simulink model "variable_delay_echo"  (R2020b)
settings: Solver=FixedStepDiscrete  StartTime=0.0  StopTime=stopTime  RelTol=1e-3
InitFcn:
  | initCallback
StopFcn:
  | stopCallback
values from neighbouring files (symbols this model uses):
  mp = sm_init_avalon_signals(mp)    [sm_callback_init.m]    (also in sm_callback_stop.m = sm_stop_verify(mp))
settings Model: Creator=Ross  LastModifiedBy=wickh
settings SolverCC: MinimalZcImpactIntegration=on
settings DataIOCC: ReturnWorkspaceOutputs=off
settings OptimizationCC: DefaultParameterBehavior=Inlined
settings DebuggingCC: ReadBeforeWriteMsg=DisableAll  WriteAfterWriteMsg=DisableAll  WriteAfterReadMsg=DisableAll  AlgebraicLoopMsg=error  MultiTaskDSMMsg=none  SingleTaskRateTransMsg=error  PregeneratedLibrarySubsystemCodeDiagnostic=none  ArithmeticOperatorsInVariantConditions=warning
settings HardwareCC: ProdBitPerPointer=32  ProdBitPerSizeT=32  ProdBitPerPtrDiffT=32  ProdLargestAtomicFloat=None  ProdIntDivRoundTo=Undefined  ProdEndianess=Unspecified  ProdWordSize=32  ProdHWDeviceType=ASIC/FPGA->ASIC/FPGA  TargetBitPerPointer=64  TargetBitPerSizeT=64  TargetBitPerPtrDiffT=64  TargetLongLongMode=on  TargetIntDivRoundTo=Zero  TargetEndianess=LittleEndian  TargetWordSize=64  TargetHWDeviceType=Custom Processor->MATLAB Host Computer  ProdEqTarget=off
settings ModelReferenceCC: UpdateModelReferenceTargets=IfOutOfDate
settings SFSimCC: SFSimEcho=off  SimUseLocalCustomCode=off  CustomCodeUndefinedFunction=UseInterfaceOnly
settings RTWCC: RTWUseLocalCustomCode=off

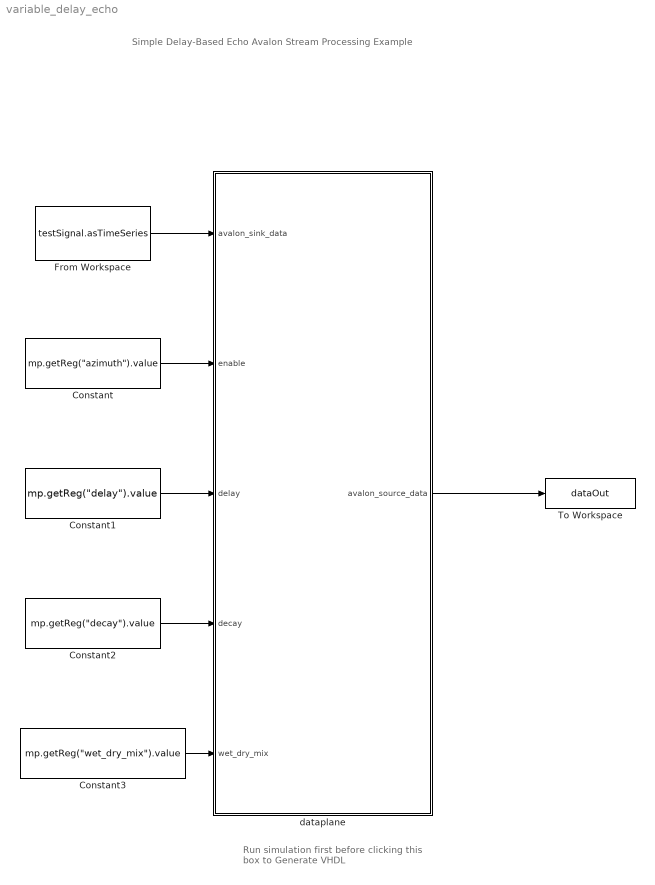
== system variable_delay_echo ==
  note: Simple Delay-Based Echo
      | Avalon Stream Processing Example
  note: Run simulation first
      | before clicking this box to
      | Generate VHDL
  Constant : Constant  Value="mp.getReg(\"azimuth\").value"  SampleTime=-1
  Constant1 : Constant  Value="mp.getReg(\"delay\").value"  SampleTime=-1
  Constant2 : Constant  Value="mp.getReg(\"decay\").value"  SampleTime=-1
  Constant3 : Constant  Value="mp.getReg(\"wet_dry_mix\").value"  SampleTime=-1
  From Workspace : FromWorkspace  VariableName=testSignal.asTimeSeries  SampleTime=mp.Ts_sim  OutputAfterFinalValue=Setting to zero
  To Workspace : ToWorkspace  VariableName=dataOut  SaveFormat=Timeseries  SampleTime=-1
  dataplane : Subsystem  TreatAsAtomicUnit=on
  wires:
  From Workspace/1 -> dataplane/1(avalon_sink_data)
  dataplane/1(avalon_source_data) -> To Workspace/1
  Constant2/1 -> dataplane/4(decay)
  Constant3/1 -> dataplane/5(wet_dry_mix)
  Constant1/1 -> dataplane/3(delay)
  Constant/1 -> dataplane/2(enable)

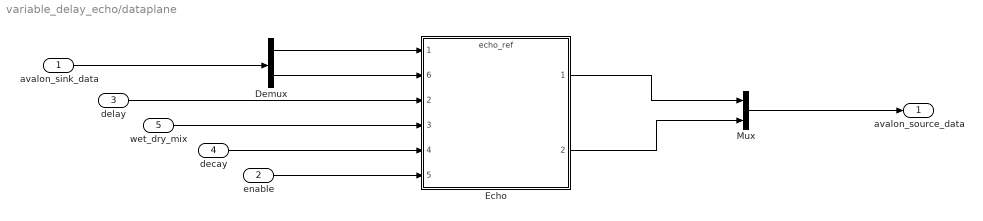
== system variable_delay_echo/dataplane ==
  avalon_sink_data : Inport
  enable : Inport  Port=2
  delay : Inport  Port=3
  decay : Inport  Port=4
  wet_dry_mix : Inport  Port=5
  Demux : Demux  Outputs=2
  Echo : ModelReference  ModelNameDialog=echo_ref  SimulationMode=Normal  ModelReferenceVersion=1.168
      settings: PortSchema="{\"entries\":[{\"content\":{\"sides\":[{\"content\":{\"connectorIds\":[\"In1\",\"In6\",\"In2\",\"In3\",\"In4\",\"In5\"]},\"type\":\"ConnectorPlacement.EquallySpacedRectSide\",\"uuid\":\"e306e1ad-d1b8-4582-952d-4c4191a99a81\"},{\"content\":{\"connectorIds\":[\"Out1\",\"Out2\"],\"side\":\"RIGHT\"},\"type\":\"ConnectorPlacement.EquallySpacedRectSide\",\"uuid\":\"8133f08a-39d0-44da-b52e-b96b1c72783c\"},{\"content\":{\"connectorIds\":[],\"side\":\"TOP\"},\"type\":\"ConnectorPlacement.EquallySpacedRectSide\",\"uuid\":\"327e31c7-8f91-4124-82a4-b2c62ce56765\"},{\"content\":{\"connectorIds\":[],\"side\":\"HIDDEN\"},\"type\":\"ConnectorPlacement.EquallySpacedRectSide\",\"uuid\":\"f85fe833-603d-4d04-9a61-60dde0930239\"}]},\"type\":\"ConnectorPlacement.EquallySpacedConnector\",\"uuid\":\"c6b2a458-4634-4ce8-98bc-50a2a0ff1bc4\"}],\"packageUris\":[\"http://schema.mathworks.com/mf0/Connector/R2020b\"],\"version\":\"1.0\"}"
  Mux : Mux  Inputs=2
  avalon_source_data : Outport  VectorParamsAs1DForOutWhenUnconnected=off
  wires:
  avalon_sink_data/1 -> Demux/1
  delay/1 -> Echo/2
  wet_dry_mix/1 -> Echo/3
  decay/1 -> Echo/4
  enable/1 -> Echo/5
  Demux/1 -> Echo/1
  Demux/2 -> Echo/6
  Echo/1 -> Mux/1
  Echo/2 -> Mux/2
  Mux/1 -> avalon_source_data/1
